simulink model "Bitwise_Calc"  (R2021a)
settings: Solver=FixedStepDiscrete  StartTime=0.0  StopTime=10.0  RelTol=1e-3  EnableMultiTasking=on
libraries: simulink x6
settings Model: Creator=Osman  LastModifiedBy=Osman
settings DataIOCC: ReturnWorkspaceOutputs=off
settings OptimizationCC: DefaultParameterBehavior=Inlined  InlineInvariantSignals=on  EnableMemcpy=off  LifeSpan=1  EfficientTunableParamExpr=on
settings DebuggingCC: UnderspecifiedInitializationDetection=Classic  MergeDetectMultiDrivingBlocksExec=none  SFMachineParentedDataDiag=warning  ArithmeticOperatorsInVariantConditions=warning
settings ModelReferenceCC: PropagateSignalLabelsOutOfModel=off
settings SFSimCC: MATLABDynamicMemAlloc=off  CustomCodeUndefinedFunction=UseInterfaceOnly
settings RTWCC: SystemTargetFile=ert.tlc  GenCodeOnly=on  TemplateMakefile=ert_default_tmf  GenerateReport=on  IncludeHyperlinkInReport=on  LaunchReport=on  GenerateTraceInfo=on  GenerateTraceReport=on  GenerateTraceReportSl=on  GenerateTraceReportSf=on  GenerateTraceReportEml=on
settings CodeAppCC: ForceParamTrailComments=on  IgnoreCustomStorageClasses=off  OperatorAnnotations=on  SimulinkDataObjDesc=on  SFDataObjDesc=on  MATLABFcnDesc=on  InsertBlockDesc=on  StateflowObjectComments=on  MATLABSourceComments=on
settings ERTTargetCC: MultiwordLength=2048  GenerateSampleERTMain=on  InlinedParameterPlacement=NonHierarchical  ERTCustomFileTemplate=example_file_process.tlc

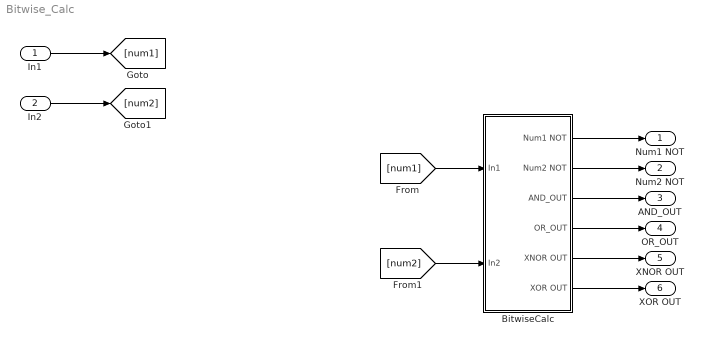
== system Bitwise_Calc ==
  In1 : Inport  OutDataTypeStr=uint32
  In2 : Inport  Port=2  OutDataTypeStr=uint32
  BitwiseCalc : Subsystem
  Num1 NOT : Outport
  Num2 NOT : Outport  Port=2
  AND_OUT : Outport  Port=3
  OR_OUT : Outport  Port=4
  XNOR OUT : Outport  Port=5
  XOR OUT : Outport  Port=6
  wires:
  In1/1 -> [num1]
  In2/1 -> [num2]
  BitwiseCalc/1(Num1 NOT) -> Num1 NOT/1
  BitwiseCalc/2(Num2 NOT) -> Num2 NOT/1
  BitwiseCalc/3(AND_OUT) -> AND_OUT/1
  BitwiseCalc/4(OR_OUT) -> OR_OUT/1
  BitwiseCalc/5(XNOR OUT) -> XNOR OUT/1
  BitwiseCalc/6(XOR OUT) -> XOR OUT/1
  [num1] -> BitwiseCalc/1(In1)
  [num2] -> BitwiseCalc/2(In2)

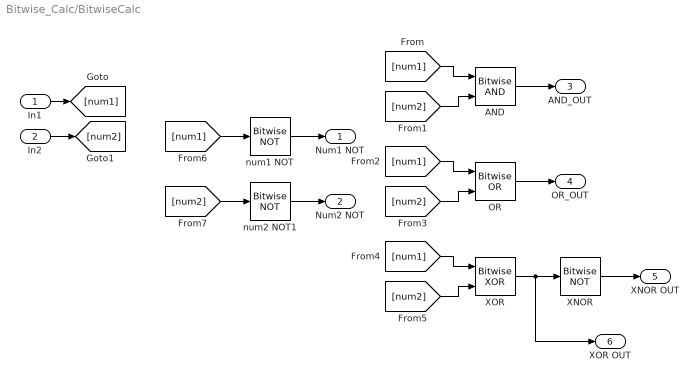
== system Bitwise_Calc/BitwiseCalc ==
  In1 : Inport  OutDataTypeStr=uint32
  In2 : Inport  Port=2  OutDataTypeStr=uint32
  AND : simulink/Logic and Bit Operations/Bitwise Operator  logicop=AND  UseBitMask=off  NumInputPorts=2  BitMask=bin2dec('11011001')  BitMaskRealWorld=Stored Integer
  OR : simulink/Logic and Bit Operations/Bitwise Operator  logicop=OR  UseBitMask=off  NumInputPorts=2  BitMask=bin2dec('11011001')  BitMaskRealWorld=Stored Integer
  XNOR : simulink/Logic and Bit Operations/Bitwise Operator  logicop=NOT  UseBitMask=off  BitMask=bin2dec('11011001')  BitMaskRealWorld=Stored Integer
  XOR : simulink/Logic and Bit Operations/Bitwise Operator  logicop=XOR  UseBitMask=off  NumInputPorts=2  BitMask=bin2dec('11011001')  BitMaskRealWorld=Stored Integer
  num1 NOT : simulink/Logic and Bit Operations/Bitwise Operator  logicop=NOT  UseBitMask=off  BitMask=bin2dec('11011001')  BitMaskRealWorld=Stored Integer
  num2 NOT1 : simulink/Logic and Bit Operations/Bitwise Operator  logicop=NOT  UseBitMask=off  BitMask=bin2dec('11011001')  BitMaskRealWorld=Stored Integer
  Num1 NOT : Outport
  Num2 NOT : Outport  Port=2
  AND_OUT : Outport  Port=3
  OR_OUT : Outport  Port=4
  XNOR OUT : Outport  Port=5
  XOR OUT : Outport  Port=6
  wires:
  num2 NOT1/1 -> Num2 NOT/1
  [num2] -> OR/2
  AND/1 -> AND_OUT/1
  [num1] -> OR/1
  [num2] -> AND/2
  [num1] -> AND/1
  [num2] -> XOR/2
  [num1] -> XOR/1
  [num2] -> num2 NOT1/1
  XOR/1 -> XOR OUT/1, XNOR/1
  [num1] -> num1 NOT/1
  OR/1 -> OR_OUT/1
  XNOR/1 -> XNOR OUT/1
  num1 NOT/1 -> Num1 NOT/1
  In1/1 -> [num1]
  In2/1 -> [num2]
